simulink model "vehicle_hostmodel_2023a_RR"  (R2023a)
settings: Solver=VariableStepAuto  StartTime=0  StopTime=1000  FixedStep=0.01  RelTol=1e-3
model workspace (MAT data in the model file):
  finalint = 0
  firstWarning = 1
  originalScenarioChecksum = '114339432DE22364D47BB28FC96DC10C'
undefined symbols (not defined in the file): Acceleration, ActorID, AngularVelocity, curvature, DefaultGear, Defined, DEND_B, DEND_S, DEND_T, direction, DiscIntNeverNeededParam, driving, Ego, gradbp, L, Lane, LF, LR, m, matlabshared, MAX_BRAKE, MAX_STEER, MAX_TORQUE, maxNumActors, MCAR, MIN_BRAKE, MIN_STEER, MIN_TORQUE, n, NUMD_B, NUMD_S, NUMD_T, Pitch, Pose, Position, psi_o, R, Roll, RRdamp, SceneInfo, session, sigbuilder_block, STEER_RATIO, stopSign_ID, Tdead, thetaRefs, TL_ID, TrackWidth, ts, Ts, User, Vdead, Velocity, WB, X_o, xRef2s, Y_o, Yaw, yRef2s
libraries: drivingscenarioandsensors x13, roadrunnerscenario x11, simulink x8, simulink_extras x5, drivingvehiclecontroller x2, trackingutilitieslib x2, robotalgslib x1, mpcadaslib x1, slpidlib x1, drivinglib x1, autolibshared x1, vehdynlibviscommon x1
(part 3 of 4)

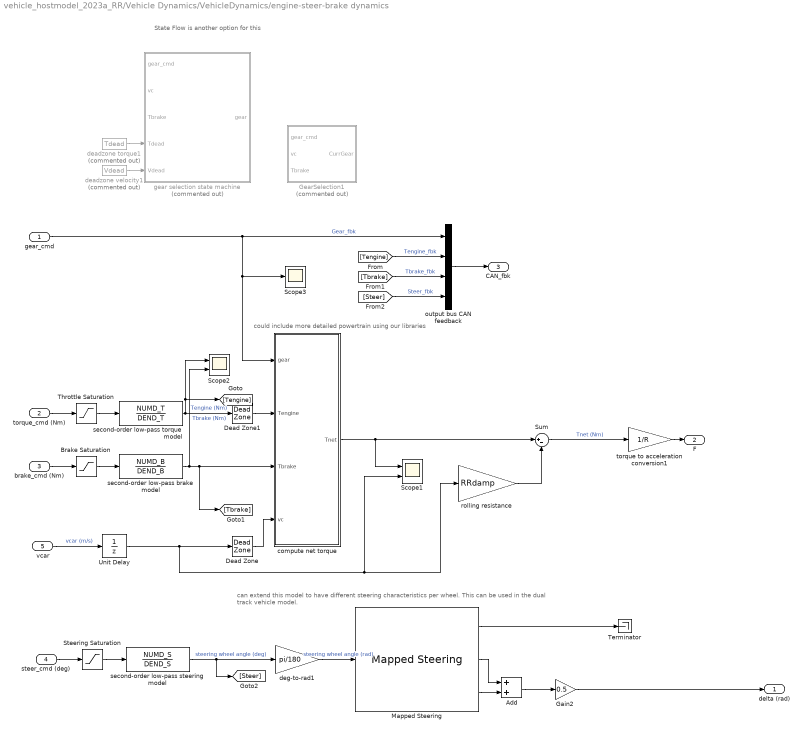
== system vehicle_hostmodel_2023a_RR/Vehicle Dynamics/VehicleDynamics/engine-steer-brake dynamics ==
  note: State Flow is another option for this
  note: could include more detailed powertrain using our libraries
  note: can extend this model to have different steering characteristics per wheel. This can be used in the dual track vehicle model.
  gear_cmd : Inport
  torque_cmd (Nm) : Inport  Port=2
  brake_cmd (Nm) : Inport  Port=3
  steer_cmd (deg) : Inport  Port=4
  vcar : Inport  Port=5
  Add : Sum
  Brake Saturation : Saturate  UpperLimit=MAX_BRAKE  LowerLimit=MIN_BRAKE
  Dead Zone : DeadZone  LowerValue=-Vdead  UpperValue=Vdead
  Dead Zone1 : DeadZone  LowerValue=-Tdead  UpperValue=Tdead
  Gain2 : Gain  Gain=0.5
  GearSelection1 : Stateflow chart  Commented=on  TreatAsAtomicUnit=on  SystemSampleTime=ts
      settings: PortSchema="{\"entries\":[{\"content\":{\"sides\":[{\"content\":{\"connectorIds\":[\"In3\",\"In2\",\"In1\"]},\"type\":\"ConnectorPlacement.EquallySpacedRectSide\",\"uuid\":\"465e5722-891f-481b-b3b6-2b8339e8e743\"},{\"content\":{\"connectorIds\":[\"Out1\"],\"side\":\"RIGHT\"},\"type\":\"ConnectorPlacement.EquallySpacedRectSide\",\"uuid\":\"28ef13cd-41d9-4e2e-8cd9-9157abf573a9\"},{\"content\":{\"connectorIds\":[],\"side\":\"TOP\"},\"type\":\"ConnectorPlacement.EquallySpacedRectSide\",\"uuid\":\"44f19923-60ae-466f-ad2a-756f1033b52e\"},{\"content\":{\"connectorIds\":[],\"side\":\"HIDDEN\"},\"type\":\"ConnectorPlacement.EquallySpacedRectSide\",\"uuid\":\"d5a146f0-4328-42be-94e3-09f51634e7da\"}]},\"type\":\"ConnectorPlacement.EquallySpacedConnector\",\"uuid\":\"14e271af-3da2-4f7d-9688-fcc3c9792006\"}],\"packageUris\":[\"http://schema.mathworks.com/mf0/Connector/R2020b\"],\"version\":\"1.0\"}"
  Mapped Steering : vehdynlibsteering/Mapped Steering  SpdDpd=off  IndexType=Steering wheel angle  GrType=Constant  StrgAngBpts=[-1.5*pi 1.5*pi]  RackDispBpts=[-40 -19.2 -4.53 4.53 19.2 40]  Gr=8.28*2*pi  GrTbl=[9.87 9.87 7.16 7.16 9.87 9.87]*2*pi  WhlLftTbl=[-1.5*pi 1.5*pi]*STEER_RATIO  WhlRghtTbl=[-1.5*pi 1.5*pi]*STEER_RATIO  VehSpdBpts=[-1 1]  SpdFctTbl=[1 1]  aMode=2
  Scope1 : Scope  NumInputPorts=2
  Scope2 : Scope  NumInputPorts=2
  Scope3 : Scope
  Steering Saturation : Saturate  UpperLimit=MAX_STEER  LowerLimit=MIN_STEER
  Sum : Sum  Inputs=|+-
  Terminator : Terminator
  Throttle Saturation : Saturate  UpperLimit=MAX_TORQUE  LowerLimit=MIN_TORQUE
  Unit Delay : UnitDelay  SampleTime=-1  HasFrameUpgradeWarning=on
  compute net torque : MATLAB Function  TreatAsAtomicUnit=on  SystemSampleTime=ts
  deadzone torque1 : Constant  Commented=on  Value=Tdead  SampleTime=ts
  deadzone velocity1 : Constant  Commented=on  Value=Vdead  SampleTime=ts
  deg-to-rad1 : Gain  Gain=pi/180
  gear selection state machine : MATLAB Function  Commented=on  TreatAsAtomicUnit=on  SystemSampleTime=ts
  output bus CAN feedback : BusCreator  Inputs=4
  rolling resistance : Gain  Gain=RRdamp
  second-order low-pass brake model : DiscreteTransferFcn  Numerator=NUMD_B  Denominator=DEND_B  SampleTime=ts
  second-order low-pass steering model : DiscreteTransferFcn  Numerator=NUMD_S  Denominator=DEND_S  SampleTime=ts
  second-order low-pass torque model : DiscreteTransferFcn  Numerator=NUMD_T  Denominator=DEND_T  SampleTime=ts
  torque to acceleration conversion1 : Gain  Gain=1/R
  delta (rad) : Outport  VectorParamsAs1DForOutWhenUnconnected=off
  F : Outport  Port=2  VectorParamsAs1DForOutWhenUnconnected=off
  CAN_fbk : Outport  Port=3  VectorParamsAs1DForOutWhenUnconnected=off
  wires:
  steer_cmd (deg)/1 -> Steering Saturation/1
  torque_cmd (Nm)/1 -> Throttle Saturation/1
  brake_cmd (Nm)/1 -> Brake Saturation/1
  second-order low-pass steering model/1 -> deg-to-rad1/1, [Steer]  "steering wheel angle (deg)"
  Throttle Saturation/1 -> second-order low-pass torque model/1
  Brake Saturation/1 -> second-order low-pass brake model/1
  Steering Saturation/1 -> second-order low-pass steering model/1
  vcar/1 -> Unit Delay/1  "vcar (m/s)"
  second-order low-pass brake model/1 -> [Tbrake], compute net torque/3(Tbrake), Scope2/2  "Tbrake (Nm)"
  second-order low-pass torque model/1 -> Dead Zone1/1, [Tengine], Scope2/1  "Tengine (Nm)"
  compute net torque/1(Tnet) -> Scope1/1, Sum/1
  rolling resistance/1 -> Sum/2
  deadzone velocity1/1 -> gear selection state machine/5(Vdead)
  deadzone torque1/1 -> gear selection state machine/4(Tdead)
  gear_cmd/1 -> output bus CAN feedback/1, Scope3/1, compute net torque/1(gear)  "Gear_fbk"
  output bus CAN feedback/1 -> CAN_fbk/1
  [Tengine] -> output bus CAN feedback/2  "Tengine_fbk"
  [Tbrake] -> output bus CAN feedback/3  "Tbrake_fbk"
  [Steer] -> output bus CAN feedback/4  "Steer_fbk"
  Mapped Steering/2 -> Add/1
  Mapped Steering/3 -> Add/2
  Add/1 -> Gain2/1
  torque to acceleration conversion1/1 -> F/1
  Mapped Steering/1 -> Terminator/1
  deg-to-rad1/1 -> Mapped Steering/1  "steering wheel angle (rad)"
  Sum/1 -> torque to acceleration conversion1/1  "Tnet (Nm)"
  Dead Zone/1 -> compute net torque/4(vc)
  Dead Zone1/1 -> compute net torque/2(Tengine)
  Unit Delay/1 -> Scope1/2, rolling resistance/1, Dead Zone/1
  Gain2/1 -> delta (rad)/1

== system vehicle_hostmodel_2023a_RR/Controllers/Lateral Controllers1/Pure Pursuit Controller1/Wheel Steering Angle Formulation ==
  alpha : Inport
  Bicycle length : Constant  Value=L
  Constant : Constant  Value=2
  Divide : Product  Inputs=*/
  Lookahead distance : Constant  Value=ld
  Product : Product
  Product1 : Product
  Sine Wave : Sin  TimeSource=Use external signal  SampleTime=0
  Trigonometric Function : Trigonometry  Operator=atan
  Al : Outport
  wires:
  Sine Wave/1 -> Product1/2
  Bicycle length/1 -> Product/2
  Constant/1 -> Product/1
  Product1/1 -> Divide/1
  Product/1 -> Product1/1
  Divide/1 -> Trigonometric Function/1
  Trigonometric Function/1 -> Al/1
  alpha/1 -> Sine Wave/1
  Lookahead distance/1 -> Divide/2

== system vehicle_hostmodel_2023a_RR/Controllers/Subsystem2/Subsystem/Function-Call Subsystem ==
  CurrVelocity : Inport
  Relative Distance : Inport  Port=2
  function : TriggerPort  VariantControl=(inherit)  ShowOutputPort=on
  MATLAB Function1 : MATLAB Function  TreatAsAtomicUnit=on
  Saturation : Saturate  UpperLimit=0.3*9.8  LowerLimit=0
  BrakingAcc : Outport
  wires:
  CurrVelocity/1 -> MATLAB Function1/1(Vel)
  Relative Distance/1 -> MATLAB Function1/2(RelDist)
  MATLAB Function1/1(BrakingAcc) -> Saturation/1
  Saturation/1 -> BrakingAcc/1

== system vehicle_hostmodel_2023a_RR/Controllers/Subsystem2/Subsystem/Subsystem2 ==
  decc_cmd : Inport
  Constant1 : Constant  Value=MCAR
  Gain : Gain  Gain=1.1*MCAR
  Gain1 : Gain  Gain=1.2*0.3*2/2
  Gain2 : Gain  Gain=0.7*9.81
  Gain4 : Gain  Gain=-R/(7.05*0.8)
  Integrator : Integrator  ExternalReset=falling
  Square : Math  Operator=square
  Sum : Sum  Inputs=+++
  T_brake_cmd : Outport
  wires:
  Square/1 -> Gain1/1
  Integrator/1 -> Square/1  "v"
  Gain4/1 -> T_brake_cmd/1  "T_eng"
  Gain1/1 -> Sum/1  "F_aero"
  Gain2/1 -> Sum/2
  decc_cmd/1 -> Integrator/2, Integrator/1, Gain/1
  Sum/1 -> Gain4/1
  Gain/1 -> Sum/3
  Constant1/1 -> Gain2/1

== system vehicle_hostmodel_2023a_RR/Controllers/Subsystem2/Subsystem1/Subsystem2 ==
  acc_cmd : Inport
  decc_cmd : Inport  Port=2
  Gain : Gain  Gain=400
  Gain1 : Gain  Gain=-400
  Subsystem : Subsystem  Commented=through
  Subsystem1 : Subsystem  Commented=through
  T_eng_cmd : Outport
  brake_cmd : Outport  Port=2
  wires:
  acc_cmd/1 -> Subsystem/1(acc_cmd)
  Subsystem/1(T_eng_cmd) -> Gain/1
  decc_cmd/1 -> Subsystem1/1(decc_cmd)
  Subsystem1/1(T_brake_cmd) -> Gain1/1
  Gain/1 -> T_eng_cmd/1
  Gain1/1 -> brake_cmd/1

== system vehicle_hostmodel_2023a_RR/Environment & Data/Roadrunner Port/Initiaal State/Initialize State ==
  VehicleRuntime : Inport
  Calculate Initial States : Subsystem
  Constant : Constant  Value=0  SampleTime=0.05
  Delay : Delay  DelayLength=1  InitialCondition=1
  InitialState : Outport
  wires:
  Delay/1 -> Calculate Initial States/Trigger
  Constant/1 -> Delay/1
  Calculate Initial States/1(EgoInitialState) -> InitialState/1
  VehicleRuntime/1 -> Calculate Initial States/1(EgoRuntime)

== system vehicle_hostmodel_2023a_RR/Environment & Data/Roadrunner Port/Initiaal State/Pack Current States ==
  note: Please be aware of the sampling time
  CurrSteer : Inport
  Info : Inport  Port=2
  CurrVelocity : Inport  Port=3
  CurrYawRate : Inport  Port=4
  egoInitialState : Inport  Port=5
  Direction : Inport  Port=6
  Bus Creator : BusCreator  Inputs=5  OutDataTypeStr=Bus: BusVehicleInfo  NonVirtualBus=on
      settings: InheritFromInputs=off
  Bus Selector : BusSelector  OutputSignals=InertFrm.RearAxl.Disp.X,InertFrm.RearAxl.Disp.Y,InertFrm.Cg.Ang.psi
  Delay1 : Delay  DelayLength=1  InitialConditionSource=Input port
      settings: InputPortMap=u0,p4
  Delayed Steering System : Subsystem
  Math Function : Math  Operator=transpose  SignedPower=on
  Mux : Mux  Inputs=3
  Radians to Degrees : simulink_extras/Transformations/Radians to Degrees
  Rate Transition{1..6} (6 alike) : RateTransition  InitialCondition=-1  OutPortSampleTime=Ts
  CurrVehicleInfo : Outport  VectorParamsAs1DForOutWhenUnconnected=off
  wires:
  CurrVelocity/1 -> Rate Transition3/1  "CurrVelocity"
  CurrSteer/1 -> Delayed Steering System/1(SteerCmd)  "CurrSteer"
  Info/1 -> Bus Selector/1  "CurrPose"
  CurrYawRate/1 -> Rate Transition6/1  "CurrYawRate"
  Direction/1 -> Rate Transition5/1  "Direction"
  Delay1/1 -> CurrVehicleInfo/1
  egoInitialState/1 -> Rate Transition1/1
  Bus Creator/1 -> Delay1/1
  Rate Transition1/1 -> Delay1/2
  Rate Transition2/1 -> Bus Creator/4
  Rate Transition3/1 -> Bus Creator/2
  Rate Transition4/1 -> Bus Creator/1
  Rate Transition5/1 -> Bus Creator/5
  Rate Transition6/1 -> Bus Creator/3
  Math Function/1 -> Rate Transition4/1
  Radians to Degrees/1 -> Mux/3
  Bus Selector/1 -> Mux/1  "<X>"
  Bus Selector/2 -> Mux/2  "<Y>"
  Bus Selector/3 -> Radians to Degrees/1  "<psi>"
  Mux/1 -> Math Function/1
  Delayed Steering System/1(CurrSteer) -> Rate Transition2/1

== system vehicle_hostmodel_2023a_RR/Environment & Data/Sensors & Perception/Tracking/Subsystem1 ==
  In2 : Inport
  EgoV : Inport  Port=2
  Camera : drivingscenarioandsensors/Vision Detection Generator  SensorIndex=1  DetectorOutput=Objects only  UpdateInterval=0.1  LaneUpdateInterval=0.1  SensorLocation=[1.9 0]  Height=1.1  Yaw=0  Pitch=1  Roll=0  BusNameSource=Auto  BusName=BusObjectDetections  BusName2Source=Auto  BusName2=BusLaneDetections  MaxNumDetectionsSource=Property  MaxNumDetections=10  MaxNumLanesSource=Property  MaxNumLanes=30  DetectionCoordinates=Ego Cartesian  SimulateUsing=Interpreted execution  MaxRange=150  BoundingBoxAccuracy=5  ProcessNoiseIntensity=5  MaxSpeed=100  MaxAllowedOcclusion=0.5  MinObjectImageSize=[5 5]  DetectionProbability=0.9  FalsePositivesPerImage=0.1  MinLaneImageSize=[20 3]  LaneBoundaryAccuracy=3  HasNoise=on  InitialSeedSource=Repeatable  InitialSeed=0  UsedSeed=0  ActorProfilesSource=From Scenario Reader block  ActorProfilesParameters=driving.internal.ActorProfilesParameters  ActorProfilesExpression=[struct('ActorID',1,'ClassID',1,'Length',4.7,'Width',1.8,'Height',1.4,'OriginOffset',[-1.35 0 0],'MeshVertices',[3.7 0.9 0.857439446366782;3.7 -0.9 0.857439446366782;3.7 -0.9 0.314878892733564;3.7 0.9 0.314878892733564;3.7 0.9 0.857439446366782;2.525 0.9 0.993079584775086;2.525 -0.9 0.993079584775086;3.7 -0.9 0.857439446366782;1.82 0.72 1.4;0.41 0.72 1.4;0.41 -0.72 1.4;1.82 -0.72 1.4;-0.295 0.9 0.993079584775086;-1 0.9 0.857439446366782;-1 -0.9 0.857439446366782;-0.295 -0.9 0.993079584775086;3.7 0.9 0.857439446366782;3.7 0.9 0.314878892733564;2.525 0.9 0.314878892733564;2.525 0.9 0.993079584775086;2.525 0.9 0.993079584775086;2.525 0.9 0.314878892733564;-0.295 0.9 0.314878892733564;-0.295 0.9 0.993079584775086;-0.295 0.9 0.993079584775086;-0.295 0.9 0.314878892733564;-1 0.9 0.355570934256055;-1 0.9 0.857439446366782;2.525 0.9 0.993079584775086;-0.295 0.9 0.993079584775086;0.41 0.72 1.4;1.82 0.72 1.4;3.7 -0.9 0.857439446366782;3.7 -0.9 0.314878892733564;2.525 -0.9 0.314878892733564;2.525 -0.9 0.993079584775086;2.525 -0.9 0.993079584775086;2.525 -0.9 0.314878892733564;-0.295 -0.9 0.314878892733564;-0.295 -0.9 0.993079584775086;-0.295 -0.9 0.993079584775086;-0.295 -0.9 0.314878892733564;-1 -0.9 0.355570934256055;-1 -0.9 0.857439446366782;2.525 -0.9 0.993079584775086;-0.295 -0.9 0.993079584775086;0.41 -0.72 1.4;1.82 -0.72 1.4;-0.295 0.9 0.993079584775086;-0.295 -0.9 0.993079584775086;0.41 -0.72 1.4;0.41 0.72 1.4;2.525 -0.9 0.993079584775086;1.82 -0.72 1.4;1.82 0.72 1.4;2.525 0.9 0.993079584775086;-1 0.9 0.857439446366782;-1 0.9 0.355570934256055;-1 -0.9 0.355570934256055;-1 -0.9 0.857439446366782;3.7 0.9 0.314878892733564;3.7 -0.9 0.314878892733564;-0.295 -0.9 0.314878892733564;-0.295 0.9 0.314878892733564;-0.295 0.9 0.314878892733564;-1 0.9 0.355570934256055;-1 -0.9 0.355570934256055;-0.295 -0.9 0.314878892733564;0 -0.63 0;0 -0.87 0;0.191030206995054 -0.63 0.0601365173421445;0.191030206995054 -0.87 0.0601365173421445;0.309093367795925 -0.63 0.217575963708927;0.309093367795925 -0.87 0.217575963708927;0.309093367795925 -0.63 0.412181821758201;0.309093367795925 -0.87 0.412181821758201;0.191030206995054 -0.63 0.569621268124983;0.191030206995054 -0.87 0.569621268124983;0 -0.63 0.629757785467128;0 -0.87 0.629757785467128;-0.191030206995054 -0.63 0.569621268124983;-0.191030206995054 -0.87 0.569621268124983;-0.309093367795925 -0.63 0.412181821758201;-0.309093367795925 -0.87 0.412181821758201;-0.309093367795925 -0.63 0.217575963708927;-0.309093367795925 -0.87 0.217575963708927;-0.191030206995054 -0.63 0.0601365173421445;-0.191030206995054 -0.87 0.0601365173421445;0 -0.63 0;0 -0.87 0;0 -0.63 0;0.191030206995054 -0.63 0.0601365173421445;0.309093367795925 -0.63 0.217575963708927;0.309093367795925 -0.63 0.412181821758201;0.191030206995054 -0.63 0.569621268124983;0 -0.63 0.629757785467128;-0.191030206995054 -0.63 0.569621268124983;-0.309093367795925 -0.63 0.412181821758201;-0.309093367795925 -0.63 0.217575963708927;-0.191030206995054 -0.63 0.0601365173421445;0 -0.87 0;0.191030206995054 -0.87 0.0601365173421445;0.309093367795925 -0.87 0.217575963708927;0.309093367795925 -0.87 0.412181821758201;0.191030206995054 -0.87 0.569621268124983;0 -0.87 0.629757785467128;-0.191030206995054 -0.87 0.569621268124983;-0.309093367795925 -0.87 0.412181821758201;-0.309093367795925 -0.87 0.217575963708927;-0.191030206995054 -0.87 0.0601365173421445;0 0.87 0;0 0.63 0;0.191030206995054 0.87 0.0601365173421445;0.191030206995054 0.63 0.0601365173421445;0.309093367795925 0.87 0.217575963708927;0.309093367795925 0.63 0.217575963708927;0.309093367795925 0.87 0.412181821758201;0.309093367795925 0.63 0.412181821758201;0.191030206995054 0.87 0.569621268124983;0.191030206995054 0.63 0.569621268124983;0 0.87 0.629757785467128;0 0.63 0.629757785467128;-0.191030206995054 0.87 0.569621268124983;-0.191030206995054 0.63 0.569621268124983;-0.309093367795925 0.87 0.412181821758201;-0.309093367795925 0.63 0.412181821758201;-0.309093367795925 0.87 0.217575963708927;-0.309093367795925 0.63 0.217575963708927;-0.191030206995054 0.87 0.0601365173421445;-0.191030206995054 0.63 0.0601365173421445;0 ...(+3718 chars)],'MeshFaces',[1 2 3;3 4 1;5 6 7;7 8 5;9 10 11;11 12 9;13 14 15;15 16 13;17 18 19;19 20 17;21 22 23;23 24 21;25 26 27;27 28 25;29 30 31;31 32 29;33 34 35;35 36 33;37 38 39;39 40 37;41 42 43;43 44 41;45 46 47;47 48 45;49 50 51;51 52 49;53 54 55;55 56 53;57 58 59;59 60 57;61 62 63;63 64 61;65 66 67;67 68 65;69 71 72;72 70 69;71 73 74;74 72 71;73 75 76;76 74 73;75 77 78;78 76 75;77 79 80;80 78 77;79 81 82;82 80 79;81 83 84;84 82 81;83 85 86;86 84 83;85 87 88;88 86 85;87 89 90;90 88 87;91 92 93;91 93 94;91 94 95;91 95 96;91 96 97;91 97 98;91 98 99;91 99 100;101 102 103;101 103 104;101 104 105;101 105 106;101 106 107;101 107 108;101 108 109;101 109 110;111 113 114;114 112 111;113 115 116;116 114 113;115 117 118;118 116 115;117 119 120;120 118 117;119 121 122;122 120 119;121 123 124;124 122 121;123 125 126;126 124 123;125 127 128;128 126 125;127 129 130;130 128 127;129 131 132;132 130 129;133 134 135;133 135 136;133 136 137;133 137 138;133 138 139;133 139 140;133 140 141;133 141 142;143 144 145;143 145 146;143 146 147;143 147 148;143 148 149;143 149 150;143 150 151;143 151 152;153 155 156;156 154 153;155 157 158;158 156 155;157 159 160;160 158 157;159 161 162;162 160 159;161 163 164;164 162 161;163 165 166;166 164 163;165 167 168;168 166 165;167 169 170;170 168 167;169 171 172;172 170 169;171 173 174;174 172 171;175 176 177;175 177 178;175 178 179;175 179 180;175 180 181;175 181 182;175 182 183;175 183 184;185 186 187;185 187 188;185 188 189;185 189 190;185 190 191;185 191 192;185 192 193;185 193 194;195 197 198;198 196 195;197 199 200;200 198 197;199 201 202;202 200 199;201 203 204;204 202 201;203 205 206;206 204 203;205 207 208;208 206 205;207 209 210;210 208 207;209 211 212;212 210 209;211 213 214;214 212 211;213 215 216;216 214 213;217 218 219;217 219 220;217 220 221;217 221 222;217 222 223;217 223 224;217 224 225;217 225 226;227 228 229;227 229 230;227 230 231;227 231 232;227 232 233;227 233 234;227 234 235;227 235 236],'RCSPattern',[10 10;10 10],'RCSAzimuthAngles',[-180 180],'RCSElevationAngles',[-90 90]); struct('ActorID',2,'ClassID',7,'Length',0.7,'Width',0.2,'Height',0.1,'OriginOffset',[0 0 0],'MeshVertices',[0.35 -0.1 0.1;0.35 0.1 0.1;-0.35 0.1 0.1;-0.35 -0.1 0.1;0.35 -0.1 0;0.35 0.1 0;-0.35 0.1 0;-0.35 -0.1 0],'MeshFaces',[6 2 1;1 5 6;8 4 3;3 7 8;6 7 3;3 2 6;5 1 4;4 8 5;4 1 2;2 3 4;7 6 5;5 8 7],'RCSPattern',[10 10;10 10],'RCSAzimuthAngles',[-180 180],'RCSElevationAngles',[-90 90])]  Intrinsics=driving.internal.cameraIntrinsics('FocalLength',[800 800],'PrincipalPoint',[320 240],'ImageSize',[480 640],'RadialDistortion',[0 0],'TangentialDistortion',[0 0],'Skew',0)
  Detection Concatenation : trackingutilitieslib/Detection Concatenation  NumInputs=3  BusNameSource=Auto  BusName=BusDetectionConcatenation  SimulateUsing=Interpreted execution
  Lidar Point Cloud Generator : drivingscenarioandsensors/Lidar Point Cloud Generator  SensorIndex=2  UpdateInterval=0.1  SensorLocation=[1.5 0]  Height=1.6  Yaw=0  Pitch=0  Roll=0  DetectionCoordinates=Ego Cartesian  HasEgoVehicle=on  EgoVehicleActorID=1  HasRoadsInputPort=on  ActorProfilesSource=From Scenario Reader block  ActorProfilesVariableName=actor_profiles  MaxRange=120  RangeAccuracy=0.002  AzimuthResolution=0.16  ElevationResolution=1.25  AzimuthLimits=[-60 60]  ElevationLimits=[ -20, 20 ]  HasNoise=on
  Lidar Point Cloud Generator1 : drivingscenarioandsensors/Lidar Point Cloud Generator  SensorIndex=3  UpdateInterval=0.1  SensorLocation=[1.5 0]  Height=1.6  Yaw=0  Pitch=0  Roll=0  DetectionCoordinates=Ego Cartesian  HasEgoVehicle=on  EgoVehicleActorID=1  HasRoadsInputPort=on  ActorProfilesSource=From Scenario Reader block  ActorProfilesVariableName=actor_profiles  MaxRange=120  RangeAccuracy=0.002  AzimuthResolution=0.16  ElevationResolution=1.25  AzimuthLimits=[60 180]  ElevationLimits=[ -20, 20 ]  HasNoise=on
  Lidar Point Cloud Generator2 : drivingscenarioandsensors/Lidar Point Cloud Generator  SensorIndex=4  UpdateInterval=0.1  SensorLocation=[1.5 0]  Height=1.6  Yaw=0  Pitch=0  Roll=0  DetectionCoordinates=Ego Cartesian  HasEgoVehicle=on  EgoVehicleActorID=1  HasRoadsInputPort=on  ActorProfilesSource=From Scenario Reader block  ActorProfilesVariableName=actor_profiles  MaxRange=120  RangeAccuracy=0.002  AzimuthResolution=0.16  ElevationResolution=1.25  AzimuthLimits=[-180 -60]  ElevationLimits=[ -20, 20 ]  HasNoise=on
  Camera Detections : Outport
  Radar detections : Outport  Port=2
  wires:
  EgoV/1 -> Lidar Point Cloud Generator1/2, Lidar Point Cloud Generator/2, Lidar Point Cloud Generator2/2
  Lidar Point Cloud Generator1/1 -> Detection Concatenation/2  "Lidar Detections"
  Lidar Point Cloud Generator2/1 -> Detection Concatenation/3  "Lidar Detections"
  Detection Concatenation/1 -> Radar detections/1
  Camera/1 -> Camera Detections/1  "Camera Detections"
  In2/1 -> Camera/1, Lidar Point Cloud Generator/1, Lidar Point Cloud Generator1/1, Lidar Point Cloud Generator2/1
  Lidar Point Cloud Generator/1 -> Detection Concatenation/1  "Lidar Detections"

== system vehicle_hostmodel_2023a_RR/Environment & Data/Visualisation & Data/Positions and States /Traffic Light Sensor ==
  note: Traffic Light Sensor
  TL_id : Inport
  Bus Creator : BusCreator  Inputs=2
  LightConfiguration : Constant  Value=TrafficLightSensorModeSelection
  Traffic Light Switching Logic : Stateflow chart  TreatAsAtomicUnit=on
  TL_State : Outport
  wires:
  LightConfiguration/1 -> Traffic Light Switching Logic/1(LightConfig)
  TL_id/1 -> Traffic Light Switching Logic/2(TL_id)
  Bus Creator/1 -> TL_State/1
  Traffic Light Switching Logic/2(trafficLight) -> Bus Creator/1
  Traffic Light Switching Logic/1(TL_ID) -> Bus Creator/2

== system vehicle_hostmodel_2023a_RR/Reference Data1/Subsystem1/Subsystem2/Subsystem ==
  note: Select method to calculate theta
  Integrator : Inport
  Curvature : Lookup_n-D  NumberOfTableDimensions=1  BreakpointsForDimension1=gradbp  Table=curvature  InternalRulePriority=Speed  RndMeth=Simplest
  Direction : Lookup_n-D  NumberOfTableDimensions=1  BreakpointsForDimension1=gradbp  Table=direction  InternalRulePriority=Speed  RndMeth=Simplest
  From Workspace1 : FromWorkspace  VariableName=yRef2  SampleTime=-1
  From Workspace2 : FromWorkspace  VariableName=xRef2  SampleTime=-1
  From Workspace3 : FromWorkspace  VariableName=gradbp  SampleTime=-1
  Goto : Goto  Commented=on  GotoTag=xRef  TagVisibility=global
  Goto1 : Goto  Commented=on  GotoTag=yRef  TagVisibility=global
  Matrix Concatenate : Concatenate  Mode=Multidimensional array  ConcatenateDimension=2
  Mux : Mux  Inputs=3
  Switch Case : SwitchCase
  Theta : Subsystem  Variant=on  VariantControlMode=label  LabelModeActiveChoice=thetaLookUpTable
  X Ref : Lookup_n-D  NumberOfTableDimensions=1  BreakpointsForDimension1=gradbp  Table=xRef2s  InternalRulePriority=Speed  RndMeth=Simplest
  Y Ref : Lookup_n-D  NumberOfTableDimensions=1  BreakpointsForDimension1Source=Input port  BreakpointsForDimension1=gradbp  TableSource=Input port  Table=yRef2s  InternalRulePriority=Speed  RndMeth=Simplest
      settings: InputPortMap=u0,p221,p5
  Out1 : Outport
  Out2 : Outport  Port=2
  CurvatureO : Outport  Port=3
  DirectionO : Outport  Port=4
  finalint : Outport  Port=5
  wires:
  Direction/1 -> DirectionO/1
  Y Ref/1 -> Theta/1(y), Mux/2, Goto1/1
  Theta/1(theta) -> Mux/3
  X Ref/1 -> Theta/2(x), Mux/1, Goto/1
  Matrix Concatenate/1 -> Out1/1
  Curvature/1 -> CurvatureO/1
  Mux/1 -> Out2/1
  From Workspace1/1 -> Y Ref/2, Matrix Concatenate/2
  From Workspace2/1 -> Matrix Concatenate/1
  From Workspace3/1 -> Y Ref/3
  Integrator/1 -> Direction/1, Curvature/1, Theta/3(dis), Y Ref/1, X Ref/1

== system vehicle_hostmodel_2023a_RR/Reference Data1/Subsystem1/Subsystem3/Subsystem ==
  note: Select method to calculate theta
  xd : Inport
  yd : Inport  Port=2
  Integrator : Inport  Port=3
  Add Constant : Bias  Bias=6.5  SaturateOnIntegerOverflow=off
  Curvature : Lookup_n-D  NumberOfTableDimensions=1  BreakpointsForDimension1=gradbp  Table=curvature  InternalRulePriority=Speed  RndMeth=Simplest
  Direction : Lookup_n-D  NumberOfTableDimensions=1  BreakpointsForDimension1=gradbp  Table=direction  InternalRulePriority=Speed  RndMeth=Simplest
  From Workspace1 : FromWorkspace  VariableName=yRef2  SampleTime=-1
  From Workspace2 : FromWorkspace  VariableName=xRef2  SampleTime=-1
  From Workspace3 : FromWorkspace  VariableName=gradbp  SampleTime=-1
  Goto : Goto  Commented=on  GotoTag=xRef  TagVisibility=global
  Goto1 : Goto  Commented=on  GotoTag=yRef  TagVisibility=global
  Matrix Concatenate : Concatenate  Mode=Multidimensional array  ConcatenateDimension=2
  Mux : Mux  Inputs=3
  Theta : Subsystem  Variant=on  VariantControlMode=label  LabelModeActiveChoice=thetaLookUpTable
  X Ref : Lookup_n-D  NumberOfTableDimensions=1  BreakpointsForDimension1Source=Input port  BreakpointsForDimension1=gradbp  TableSource=Input port  Table=xRef2s  InternalRulePriority=Speed  RndMeth=Simplest
      settings: InputPortMap=u0,p221,p5
  Y Ref : Lookup_n-D  NumberOfTableDimensions=1  BreakpointsForDimension1Source=Input port  BreakpointsForDimension1=gradbp  TableSource=Input port  Table=yRef2s  InternalRulePriority=Speed  RndMeth=Simplest
      settings: InputPortMap=u0,p221,p5
  Out1 : Outport
  Out2 : Outport  Port=2
  CurvatureO : Outport  Port=3
  DirectionO : Outport  Port=4
  wires:
  Direction/1 -> DirectionO/1
  Theta/1(theta) -> Mux/3
  Matrix Concatenate/1 -> Out1/1
  Curvature/1 -> CurvatureO/1
  Mux/1 -> Out2/1
  From Workspace1/1 -> Add Constant/1, Matrix Concatenate/2
  From Workspace2/1 -> X Ref/2, Matrix Concatenate/1
  From Workspace3/1 -> Y Ref/3, X Ref/3
  X Ref/1 -> Theta/2(x), Mux/1
  Add Constant/1 -> Y Ref/2
  Y Ref/1 -> Theta/1(y), Mux/2
  Integrator/1 -> Direction/1, Curvature/1, Theta/3(dis), Y Ref/1, X Ref/1

== system vehicle_hostmodel_2023a_RR/Reference Data1/Subsystem2/Subsystem/Theta ==
  note: 1) Add Subsystem or Model blocks as valid variant choices.
      | 2) You cannot connect blocks at this level. At simulation, connectivity is automatically
      | determined, based on the active variant and port name matching.
  y : Inport
  x : Inport  Port=2
  dis : Inport  Port=3
  thetaBlocks : Subsystem  VariantControl=thetaSimulinkBlock
  thetaLt : Subsystem  VariantControl=thetaLookUpTable
  theta : Outport

== system vehicle_hostmodel_2023a_RR/Reference Data1/Subsystem3/Subsystem/Theta ==
  note: 1) Add Subsystem or Model blocks as valid variant choices.
      | 2) You cannot connect blocks at this level. At simulation, connectivity is automatically
      | determined, based on the active variant and port name matching.
  y : Inport
  x : Inport  Port=2
  dis : Inport  Port=3
  thetaBlocks : Subsystem  VariantControl=thetaSimulinkBlock
  thetaLt : Subsystem  VariantControl=thetaLookUpTable
  theta : Outport

== system vehicle_hostmodel_2023a_RR/Controllers/Subsystem2/Subsystem1/Subsystem2/Subsystem ==
  acc_cmd : Inport
  Constant1 : Constant  Value=MCAR
  Gain : Gain  Gain=1.1*MCAR
  Gain1 : Gain  Gain=1.2*0.3*2/2
  Gain2 : Gain  Gain=0.7*9.81
  Gain4 : Gain  Gain=R/(7.05*0.8)
  Integrator : Integrator  ExternalReset=falling
  Square : Math  Operator=square
  Sum : Sum  Inputs=+++
  T_eng_cmd : Outport
  wires:
  Constant1/1 -> Gain2/1
  Gain/1 -> Sum/3
  Sum/1 -> Gain4/1
  acc_cmd/1 -> Gain/1, Integrator/2, Integrator/1
  Gain2/1 -> Sum/2
  Gain1/1 -> Sum/1  "F_aero"
  Gain4/1 -> T_eng_cmd/1  "T_eng"
  Integrator/1 -> Square/1  "v"
  Square/1 -> Gain1/1

== system vehicle_hostmodel_2023a_RR/Controllers/Subsystem2/Subsystem1/Subsystem2/Subsystem1 ==
  decc_cmd : Inport
  Constant1 : Constant  Value=MCAR
  Gain : Gain  Gain=1.1*MCAR
  Gain1 : Gain  Gain=1.2*0.3*2/2
  Gain2 : Gain  Gain=0.7*9.81
  Gain4 : Gain  Gain=-R/(7.05*0.8)
  Integrator : Integrator  ExternalReset=falling
  Square : Math  Operator=square
  Sum : Sum  Inputs=+++
  T_brake_cmd : Outport
  wires:
  Square/1 -> Gain1/1
  Integrator/1 -> Square/1  "v"
  Gain4/1 -> T_brake_cmd/1  "T_eng"
  Gain1/1 -> Sum/1  "F_aero"
  Gain2/1 -> Sum/2
  decc_cmd/1 -> Integrator/2, Integrator/1, Gain/1
  Sum/1 -> Gain4/1
  Gain/1 -> Sum/3
  Constant1/1 -> Gain2/1

== system vehicle_hostmodel_2023a_RR/Environment & Data/Roadrunner Port/Initiaal State/Initialize State/Calculate Initial States ==
  EgoRuntime : Inport
  Trigger : TriggerPort  VariantControl=(inherit)  InitialTriggerSignalState=negative  PortDimensions=1
  Calculate Initial States : MATLAB Function  TreatAsAtomicUnit=on
  EgoInitialState : Outport
  wires:
  EgoRuntime/1 -> Calculate Initial States/1(egoRuntime)
  Calculate Initial States/1(egoInitialState) -> EgoInitialState/1

== system vehicle_hostmodel_2023a_RR/Environment & Data/Roadrunner Port/Initiaal State/Pack Current States/Delayed Steering System ==
  SteerCmd : Inport
  Add : Sum  Inputs=+-
  Delay : TransferFcn  Denominator=[0.1 0]
  CurrSteer : Outport  VectorParamsAs1DForOutWhenUnconnected=off
  wires:
  Add/1 -> Delay/1
  SteerCmd/1 -> Add/1
  Delay/1 -> CurrSteer/1, Add/2

== system vehicle_hostmodel_2023a_RR/Reference Data1/Subsystem1/Subsystem2/Subsystem/Theta ==
  note: 1) Add Subsystem or Model blocks as valid variant choices.
      | 2) You cannot connect blocks at this level. At simulation, connectivity is automatically
      | determined, based on the active variant and port name matching.
  y : Inport
  x : Inport  Port=2
  dis : Inport  Port=3
  thetaBlocks : Subsystem  VariantControl=thetaSimulinkBlock
  thetaLt : Subsystem  VariantControl=thetaLookUpTable
  theta : Outport

== system vehicle_hostmodel_2023a_RR/Reference Data1/Subsystem1/Subsystem3/Subsystem/Theta ==
  note: 1) Add Subsystem or Model blocks as valid variant choices.
      | 2) You cannot connect blocks at this level. At simulation, connectivity is automatically
      | determined, based on the active variant and port name matching.
  y : Inport
  x : Inport  Port=2
  dis : Inport  Port=3
  thetaBlocks : Subsystem  VariantControl=thetaSimulinkBlock
  thetaLt : Subsystem  VariantControl=thetaLookUpTable
  theta : Outport

== system vehicle_hostmodel_2023a_RR/Reference Data1/Subsystem2/Subsystem/Theta/thetaBlocks ==
  note: theta calculated from Simulink blocks
  y : Inport
  x : Inport  Port=2
  dis : Inport  Port=3
  Atan2 : Trigonometry  Operator=atan2  ApproximationMethod=CORDIC
  Difference : simulink/Discrete/Difference  ICPrevInput=0.0  OutMin=[]  OutMax=[]  OutDataType=fixdt(1, 16)  OutScaling=2^-10  DoSatur=off
  Difference1 : simulink/Discrete/Difference  ICPrevInput=0.0  OutMin=[]  OutMax=[]  OutDataType=fixdt(1, 16)  OutScaling=2^-10  DoSatur=off
  IC : InitialCondition  Value=psi_o
  Radians to Degrees : simulink_extras/Transformations/Radians to Degrees
  Terminator : Terminator
  theta : Outport
  wires:
  IC/1 -> Radians to Degrees/1
  Atan2/1 -> IC/1
  dis/1 -> Terminator/1
  x/1 -> Difference1/1
  y/1 -> Difference/1
  Radians to Degrees/1 -> theta/1
  Difference/1 -> Atan2/1
  Difference1/1 -> Atan2/2

== system vehicle_hostmodel_2023a_RR/Reference Data1/Subsystem2/Subsystem/Theta/thetaLt ==
  note: Check out the script "setUpModel" to understand how we have calculated theta
  note: theta based on lookup table
  y : Inport
  x : Inport  Port=2
  dis : Inport  Port=3
  Terminator : Terminator
  Terminator1 : Terminator
  Theta Ref : Lookup_n-D  NumberOfTableDimensions=1  BreakpointsForDimension1=gradbp  Table=thetaRefs  InternalRulePriority=Speed  RndMeth=Simplest
  theta : Outport
  wires:
  Theta Ref/1 -> theta/1
  dis/1 -> Theta Ref/1
  x/1 -> Terminator1/1
  y/1 -> Terminator/1

== system vehicle_hostmodel_2023a_RR/Reference Data1/Subsystem3/Subsystem/Theta/thetaBlocks ==
  note: theta calculated from Simulink blocks
  y : Inport
  x : Inport  Port=2
  dis : Inport  Port=3
  Atan2 : Trigonometry  Operator=atan2  ApproximationMethod=CORDIC
  Difference : simulink/Discrete/Difference  ICPrevInput=0.0  OutMin=[]  OutMax=[]  OutDataType=fixdt(1, 16)  OutScaling=2^-10  DoSatur=off
  Difference1 : simulink/Discrete/Difference  ICPrevInput=0.0  OutMin=[]  OutMax=[]  OutDataType=fixdt(1, 16)  OutScaling=2^-10  DoSatur=off
  IC : InitialCondition  Value=psi_o
  Radians to Degrees : simulink_extras/Transformations/Radians to Degrees
  Terminator : Terminator
  theta : Outport
  wires:
  IC/1 -> Radians to Degrees/1
  Atan2/1 -> IC/1
  dis/1 -> Terminator/1
  x/1 -> Difference1/1
  y/1 -> Difference/1
  Radians to Degrees/1 -> theta/1
  Difference/1 -> Atan2/1
  Difference1/1 -> Atan2/2

== system vehicle_hostmodel_2023a_RR/Reference Data1/Subsystem3/Subsystem/Theta/thetaLt ==
  note: Check out the script "setUpModel" to understand how we have calculated theta
  note: theta based on lookup table
  y : Inport
  x : Inport  Port=2
  dis : Inport  Port=3
  Terminator : Terminator
  Terminator1 : Terminator
  Theta Ref : Lookup_n-D  NumberOfTableDimensions=1  BreakpointsForDimension1=gradbp  Table=thetaRefs  InternalRulePriority=Speed  RndMeth=Simplest
  theta : Outport
  wires:
  Theta Ref/1 -> theta/1
  dis/1 -> Theta Ref/1
  x/1 -> Terminator1/1
  y/1 -> Terminator/1

== system vehicle_hostmodel_2023a_RR/Reference Data1/Subsystem1/Subsystem2/Subsystem/Theta/thetaBlocks ==
  note: theta calculated from Simulink blocks
  y : Inport
  x : Inport  Port=2
  dis : Inport  Port=3
  Atan2 : Trigonometry  Operator=atan2  ApproximationMethod=CORDIC
  Difference : simulink/Discrete/Difference  ICPrevInput=0.0  OutMin=[]  OutMax=[]  OutDataType=fixdt(1, 16)  OutScaling=2^-10  DoSatur=off
  Difference1 : simulink/Discrete/Difference  ICPrevInput=0.0  OutMin=[]  OutMax=[]  OutDataType=fixdt(1, 16)  OutScaling=2^-10  DoSatur=off
  IC : InitialCondition  Value=psi_o
  Radians to Degrees : simulink_extras/Transformations/Radians to Degrees
  Terminator : Terminator
  theta : Outport
  wires:
  IC/1 -> Radians to Degrees/1
  Atan2/1 -> IC/1
  dis/1 -> Terminator/1
  x/1 -> Difference1/1
  y/1 -> Difference/1
  Radians to Degrees/1 -> theta/1
  Difference/1 -> Atan2/1
  Difference1/1 -> Atan2/2

== system vehicle_hostmodel_2023a_RR/Reference Data1/Subsystem1/Subsystem2/Subsystem/Theta/thetaLt ==
  note: Check out the script "setUpModel" to understand how we have calculated theta
  note: theta based on lookup table
  y : Inport
  x : Inport  Port=2
  dis : Inport  Port=3
  Terminator : Terminator
  Terminator1 : Terminator
  Theta Ref : Lookup_n-D  NumberOfTableDimensions=1  BreakpointsForDimension1=gradbp  Table=thetaRefs  InternalRulePriority=Speed  RndMeth=Simplest
  theta : Outport
  wires:
  Theta Ref/1 -> theta/1
  dis/1 -> Theta Ref/1
  x/1 -> Terminator1/1
  y/1 -> Terminator/1

== system vehicle_hostmodel_2023a_RR/Reference Data1/Subsystem1/Subsystem3/Subsystem/Theta/thetaBlocks ==
  note: theta calculated from Simulink blocks
  y : Inport
  x : Inport  Port=2
  dis : Inport  Port=3
  Atan2 : Trigonometry  Operator=atan2  ApproximationMethod=CORDIC
  Difference : simulink/Discrete/Difference  ICPrevInput=0.0  OutMin=[]  OutMax=[]  OutDataType=fixdt(1, 16)  OutScaling=2^-10  DoSatur=off
  Difference1 : simulink/Discrete/Difference  ICPrevInput=0.0  OutMin=[]  OutMax=[]  OutDataType=fixdt(1, 16)  OutScaling=2^-10  DoSatur=off
  IC : InitialCondition  Value=psi_o
  Radians to Degrees : simulink_extras/Transformations/Radians to Degrees
  Terminator : Terminator
  theta : Outport
  wires:
  IC/1 -> Radians to Degrees/1
  Atan2/1 -> IC/1
  dis/1 -> Terminator/1
  x/1 -> Difference1/1
  y/1 -> Difference/1
  Radians to Degrees/1 -> theta/1
  Difference/1 -> Atan2/1
  Difference1/1 -> Atan2/2

== system vehicle_hostmodel_2023a_RR/Reference Data1/Subsystem1/Subsystem3/Subsystem/Theta/thetaLt ==
  note: Check out the script "setUpModel" to understand how we have calculated theta
  note: theta based on lookup table
  y : Inport
  x : Inport  Port=2
  dis : Inport  Port=3
  Terminator : Terminator
  Terminator1 : Terminator
  Theta Ref : Lookup_n-D  NumberOfTableDimensions=1  BreakpointsForDimension1=gradbp  Table=thetaRefs  InternalRulePriority=Speed  RndMeth=Simplest
  theta : Outport
  wires:
  Theta Ref/1 -> theta/1
  dis/1 -> Theta Ref/1
  x/1 -> Terminator1/1
  y/1 -> Terminator/1

== matlab function vehicle_hostmodel_2023a_RR/Environment & Data/Roadrunner Port/ENU to NWD/MATLAB Function2 ==
  data: u input; y output; y1 output
function [y,y1] = fcn(u)

y = u(:,1);
y1=u(:,2);

== matlab function vehicle_hostmodel_2023a_RR/Environment & Data/Roadrunner Port/ENU to NWD/2D RefWaypoints ==
  data: u input; y output
function y = fcn(u)

y = u(:,1:2);
end

== matlab function vehicle_hostmodel_2023a_RR/Controllers/Subsystem2/MATLAB Function ==
  data: u input; accel output; decel output
function [accel, decel] = fcn(u)
if(u>0)
    accel=u; decel=0;
elseif(u<0)
    accel=0; decel=-u;
else
    accel=0;decel=0;
end

== matlab function vehicle_hostmodel_2023a_RR/Controllers/Subsystem2/Subsystem/Desired Velocity Profile ==
  data: MaxBrakeFlag output; CurrVel input; DesiredDecel output; RelDist input; Dist1 output; StoppingDist input
function [MaxBrakeFlag,DesiredDecel,Dist1] = VelocityProfile(CurrVel,RelDist,StoppingDist)
% time remaining = (current velocity) / (deceleration).
% desired velocity = (stopping distance - current distance) / time remaining.
Dist1 = RelDist - (2.6850+1);
Dist = Dist1 - StoppingDist;
if Dist1 <= 2
    MaxBrakeFlag = 1;
    DesiredDecel = 0;
else
    MaxBrakeFlag = 0;
    DesiredDecel = min((CurrVel^2)/(2*Dist),3.5);
end
%     Dist = RelDist - (2.6850 + 3);
%     Decel = (CurrVel^2)/(2*Dist);
%     RemainingTime = CurrVel/Decel;
%     DesiredVel = Dist/RemainingTime; % DesiredVel = CurrVel/2

== matlab function vehicle_hostmodel_2023a_RR/Controllers/Subsystem2/Subsystem/Function-Call Subsystem/MATLAB Function1 ==
  data: Vel input; BrakingAcc output; RelDist input
function BrakingAcc = fcn(Vel,RelDist)

DistOffset = 1;
Dist = RelDist - DistOffset;
BrakingAcc = (Vel^2)/(2*Dist);

== matlab function vehicle_hostmodel_2023a_RR/Environment & Data/Visualisation & Data/Positions and States /MATLAB Function2 ==
  data: Actors input; ss_poses output; ss_State input

function ss_poses = findssposes(Actors, ss_State)

n=length(ss_State);
ss_poses=zeros(n,4);
indices=zeros(n,1);
ID=zeros(length(Actors),1);

for i=1:length(Actors)
 ID(i)=Actors(i).ActorID;
end

indices=find(ismember(ID,ss_State));
if(~isempty(indices))
    
    for i=1:n
        ss_poses(i,:)=([Actors(indices(i)).Position(:)',ss_State(i)]);
    end
end

ss_poses(ss_poses==0)=NaN;






% ss1_poses=zeros(1,4);
% ss2_poses=zeros(1,4);
% for i=1:length(Actors)
%     ID=Actors(i).ActorID;
%     
%     if(ID==ss1_State(1))
%         ss1_poses=[Actors(i).Position(:)',ss1_State(1)];
%     elseif ID== (ss1_State(2))
%         ss2_poses=[Actors(i).Position(:)',ss1_State(2)];
%     
%     end
%   
% end
% ss1_poses(ss1_poses==0)=NaN;   
% ss2_poses(ss2_poses==0)=NaN;

== matlab function vehicle_hostmodel_2023a_RR/Environment & Data/Visualisation & Data/Positions and States /MATLAB Function1 ==
  data: Actors input; TL_poses output; TL_State input

function TL_poses = findTLposes(Actors, TL_State)
n=length(TL_State);
TL_poses=zeros(n/2,5);
indices=zeros(n/2,1);
ID=zeros(length(Actors),1);

for i=1:length(Actors)
 ID(i)=Actors(i).ActorID;
end

indices=find(ismember(ID,TL_State(n/2+1:end)));
if (~isempty(indices))

    for i=1:n/2
        TL_poses(i,:)=([Actors(indices(i)).Position(:)',TL_State(i),ID(indices(i))]);

    end
end
TL_poses(TL_poses==0)=NaN;

== stateflow chart vehicle_hostmodel_2023a_RR/Environment & Data/Visualisation & Data/Positions and States /Traffic Light Sensor/Traffic Light Switching Logic ==
  state STEADYRED
    entry:
    trafficLight(:)= Red; TL_ID=TL_id;
  state STEADYGREEN
    entry:
    trafficLight(:)= Green; TL_ID=TL_id;
  state START
    entry:
    trafficLight=TL_id;
    trafficLight(:)= Black;TL_ID=TL_id;
  state TRAFFICLIGHT_ODDYELLOW_EVENRED
    entry:
    trafficLight(1:2:end)=Yellow;TL_ID(1:2:end)=TL_id(1:2:end);
    trafficLight(2:2:end) = Red;TL_ID(2:2:end)=TL_id(2:2:end);
  state TRAFFICLIGHT_ODDGREEN_EVENRED
    entry:
    trafficLight(1:2:end)=Green;TL_ID(1:2:end)=TL_id(1:2:end);
    trafficLight(2:2:end) = Red;TL_ID(2:2:end)=TL_id(2:2:end);
  state TRAFFICLIGHT_ODDRED_EVENYELLOW
    entry:
    trafficLight(1:2:end)=Red;TL_ID(1:2:end)=TL_id(1:2:end);
    trafficLight(2:2:end) = Yellow;TL_ID(2:2:end)=TL_id(2:2:end);
  state TRAFFICLIGHT_ODDRED_EVENGREEN
    entry:
    trafficLight(1:2:end)=Red;TL_ID(1:2:end)=TL_id(1:2:end);
    trafficLight(2:2:end) = Green;TL_ID(2:2:end)=TL_id(2:2:end);
  (default) -> START
  START -> STEADYGREEN [order 3] : [LightConfig==1]
  START -> STEADYRED [order 1] : [LightConfig==2]
  START -> TRAFFICLIGHT_ODDGREEN_EVENRED [order 2] : [LightConfig ==3]
  TRAFFICLIGHT_ODDGREEN_EVENRED -> TRAFFICLIGHT_ODDYELLOW_EVENRED : after(4,sec)
  TRAFFICLIGHT_ODDYELLOW_EVENRED -> TRAFFICLIGHT_ODDRED_EVENGREEN : after(1,sec)
  TRAFFICLIGHT_ODDRED_EVENYELLOW -> TRAFFICLIGHT_ODDGREEN_EVENRED : after(1,sec)
  TRAFFICLIGHT_ODDRED_EVENGREEN -> TRAFFICLIGHT_ODDRED_EVENYELLOW : after(4,sec)
  data: Green constant double =3; Red constant double =1; Yellow constant double =2; LightConfig input; TL_id input; Black constant double =0; TL_ID output; trafficLight output

== matlab function vehicle_hostmodel_2023a_RR/Environment & Data/Sensors & Perception/MATLAB Function ==
  data: SceneID output; ObjRelVel output; SceneRelVel output; SceneDist output; ObjectDist output; ObjAhead output; SDist input; Tracking input; SceneAhead output; RelVelmin output; RelDistmin output; Trans input; ObjectMIO_Position output; ObjTracks output; SceneTracks output
function [SceneID,ObjRelVel,SceneRelVel,SceneDist,ObjectDist,ObjAhead,SceneAhead,RelVelmin,RelDistmin,ObjectMIO_Position,ObjTracks,SceneTracks]= SFDetections(SDist,Tracking, Trans)
ObjectID = zeros(20,1);
TrackPos = zeros(3,20);
TrackVel = zeros(3,20);
ObjTracks = zeros(6,20);
SceneTracks = zeros(6,20);
ObjectDist = 100; % zeros(20,1);
SceneDist = 100;
ObjRelVel = 10;
SceneRelVel = 10;
% ScenePos = [0 0];
ObjAhead = 0;
SceneAhead = 0;
SceneID = 0;
TracksNum = 0;
ObjectMIO_Position = zeros(3,1);
s1 = 0;
s2 = 0;

% Tracks from sensors
% TracksNum = Tracking.NumTracks;

% Ground truth
TracksNum1 = Tracking.NumActors;
% reading only tracks in the field of view (180 deg)
for k = 1:TracksNum1
    ang = atan2d(Tracking.Actors(k).Position(2),Tracking.Actors(k).Position(1));
    if abs(ang) < 90
        TracksNum = TracksNum + 1;
        ObjectID(TracksNum) = Tracking.Actors(k).ActorID;
        TrackPos(:,TracksNum) = Tracking.Actors(k).Position;
        TrackVel(:,TracksNum) = Tracking.Actors(k).Velocity;
    end
end


for t = 1:TracksNum
    % Tracks from sensors
    % ObjectID(t) = Tracking.Tracks(t).ObjectAttributes.TargetIndex; % .ObjectClassID;
    % TrackPos(:,t) = Tracking.Tracks(t).State(1:2:5);
    % TrackVel(:,t) = Tracking.Tracks(t).State(2:2:6);

    % % Ground truth
    % ObjectID(t) = Tracking.Actors(t).ActorID;
    % TrackPos(:,t) = Tracking.Actors(t).Position;
    % TrackVel(:,t) = Tracking.Actors(t).Velocity;

    % All objects and scene Detections

    if ObjectID(t) > 9 % for roadrunner SS scene
        ObjectID(t) = 7;
    end

    if ObjectID(t) == 7 % Scenes: 7=SS 8=TL 9=RA 10=RRC % labels {1,2,3,4} => {'TrafficLight','StopSign','RailRoadCrossing','RoundAbout'};
        s1 = s1 + 1;
        % Tracks from sensors
        % SceneTracks(:,s1) = Tracking.Tracks(t).State(:);

        % Ground Truth
        SceneTracks(:,s1) = [TrackPos(1,t) TrackVel(1,t) TrackPos(2,t) TrackVel(2,t) TrackPos(3,t) TrackVel(3,t)]';
    elseif ObjectID(t) < 7 && ObjectID(t) > 0 % Objects
        s2 = s2 + 1;
        % Tracks from sensors
        % ObjTracks(:,s2) = Tracking.Tracks(t).State(:);

        % Ground Truth
        ObjTracks(:,s2) = [TrackPos(1,t) TrackVel(1,t) TrackPos(2,t) TrackVel(2,t) TrackPos(3,t) TrackVel(3,t)]';
    end
   




    if TrackPos(2,t) < 2 && TrackPos(2,t) > -6 && abs(TrackPos(1,t)) <= SDist
        
        if ObjectID(t) >= 7 && Trans ~= 1 % 7=SS 8=TL 9=RA 10=RRC % labels {1,2,3,4} => {'TrafficLight','StopSign','RailRoadCrossing','RoundAbout'};
            SceneAhead = 1;
            SceneDist = min(SceneDist,TrackPos(1,t));
            if TrackPos(1,t) <= SceneDist
                % ScenePos = TrackPos(1:2,t)';
                SceneRelVel = TrackVel(1,t);
                SceneID = ObjectID(t);
            end
        end

        if ObjectID(t) < 7 && ObjectID(t) > 0
            ObjAhead = 1;
            ObjectDist = min(ObjectDist,TrackPos(1,t));
            ObjectMIO_Position(:,1) = TrackPos(:,t);

            if TrackPos(1,t) <= ObjectDist
                ObjRelVel = TrackVel(1,t);
                ObjID = ObjectID(t);
            end
        end

    end
    
end

if Trans == 1  % ObjectDist <= SceneDist
    RelVelmin = ObjRelVel;
    RelDistmin = ObjectDist;
else
    RelVelmin = min(SceneRelVel,ObjRelVel);
    RelDistmin = min(SceneDist,ObjectDist);
end

== matlab function vehicle_hostmodel_2023a_RR/Vehicle Dynamics/Info2ActorState/MATLAB Function ==
  data: X input; Position output; Y input; Z input
function Position = fcn(X, Y, Z)

Position = [X Y, Z];

== matlab function vehicle_hostmodel_2023a_RR/Subsystem/PathPlanner/MATLAB Function4 ==
  data: Distance output; output input; CurrentPose input; point output
function [Distance,point] = d2f(output,CurrentPose)



%Distance = norm(output(end,:) - CurrentPose(1:2)');
Distance= output(end,1)- CurrentPose(1);
point=output(end,:);

end

%Distance = sqrt(CurrentPose(1)-output(99,1))^2 + (CurrentPose(2)-output(99,2)^2);
%CurrentPose
%output=zeros(99,2);
%lastPoint = output(end,:);
%dx = lastPoint(1) - x;
%dx= output(end,1)-x;
%dy = output(end,2) - y;
%distance = sqrt(dx^2 + dy^2);
